simulink subsystem "TurtlebotPlant"  (R2021b)
settings: Solver=VariableStepAuto  StartTime=0.0  StopTime=10.0  RelTol=1e-3
values from neighbouring files (symbols this model uses):
  x0 = [0;0;0]    [config.m]
settings Model: Creator=delur  LastModifiedBy=delur

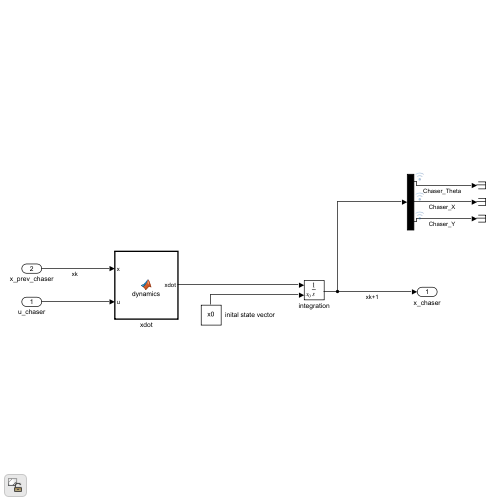
[thumbnail: Simulink's stored preview of the top-level diagram]
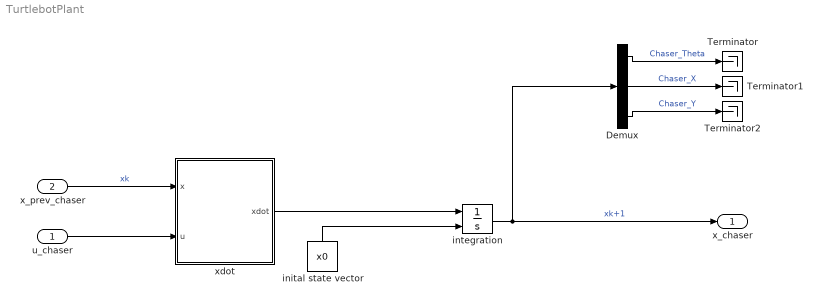
== system TurtlebotPlant ==
  u_chaser : Inport
  x_prev_chaser : Inport  Port=2
  Demux : Demux  Outputs=3
  Terminator : Terminator
  Terminator1 : Terminator
  Terminator2 : Terminator
  inital state vector : Constant  Value=x0
  integration : Integrator  InitialConditionSource=external
  xdot : MATLAB Function  TreatAsAtomicUnit=on
  x_chaser : Outport
  wires:
  u_chaser/1 -> xdot/2(u)
  integration/1 -> x_chaser/1, Demux/1  "xk+1"
  x_prev_chaser/1 -> xdot/1(x)  "xk"
  xdot/1(xdot) -> integration/1
  inital state vector/1 -> integration/2
  Demux/2 -> Terminator1/1  "Chaser_X"
  Demux/3 -> Terminator2/1  "Chaser_Y"
  Demux/1 -> Terminator/1  "Chaser_Theta"

== matlab function TurtlebotPlant/xdot ==
  data: x input; u input; xdot output
function xdot = dynamics(x,u)
% STATE VECTOR X: [theta,x,y], [orientation, x pos inertial, y pos inertial
% (pose state)
% CONTROL INPUT u: [uw,uv], [angular rate, linear velocity] (twist control)
xdot = zeros(3,1);

xdot(1) = u(1); % theta_dot
xdot(2) = u(2)*cos(x(1)); %x inertial velocity
xdot(3) = u(2)*sin(x(1)); %y inertial velocity

end
